simulink model "Motor1conCorrientePrevia"  (R2025b)
settings: Solver=FixedStepDiscrete  StartTime=0.0  StopTime=inf  FixedStep=0.01  RelTol=1e-3  EnableMultiTasking=on
libraries: arduinolib x7, simulink x5, arduinosensorlib x1
settings Model: SimulationMode=external  ExtModeTrigDuration=2  Creator=Vizca  LastModifiedBy=josee
settings SolverCC: AutoInsertRateTranBlk=on
settings OptimizationCC: EnhancedBackFolding=on  PassReuseOutputArgsAs=Individual arguments  ZeroExternalMemoryAtStartup=off  ZeroInternalMemoryAtStartup=off  MaxStackSize=64  OptimizeBlockOrder=speed  DifferentSizesBufferReuse=on  OptimizationCustomize=off  EfficientTunableParamExpr=on
settings DebuggingCC: ParameterTunabilityLossMsg=error
settings HardwareCC: ProdBitPerInt=16.0  ProdBitPerPointer=16.0  ProdBitPerSizeT=16.0  ProdBitPerPtrDiffT=16.0  ProdLargestAtomicFloat=None  ProdWordSize=8.0  ProdHWDeviceType=Atmel->AVR
settings RTWCC: SystemTargetFile=ert.tlc  HardwareBoard=Arduino Uno  TemplateMakefile=ert_default_tmf  Toolchain=Arduino AVR  BuildConfiguration=Faster Runs  Description=Embedded Coder
settings CodeAppCC: ForceParamTrailComments=on  IgnoreCustomStorageClasses=off  OperatorAnnotations=on  SimulinkDataObjDesc=on  SFDataObjDesc=on  InsertBlockDesc=on
settings ERTTargetCC: ExtModeTransport=3.0  ExtModeStaticAlloc=on  ExtModeAutomaticAllocSize=off  ExtModeStaticAllocSize=250.0  ExtModeMexFile=ext_xcp  ExtModeIntrfLevel=Level2 - Open  InlinedParameterPlacement=Hierarchical  SupportContinuousTime=on  SupportVariableSizeSignals=on

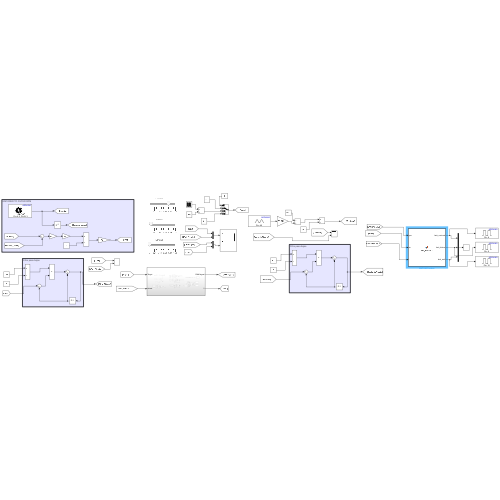
[thumbnail: Simulink's stored preview of the top-level diagram]
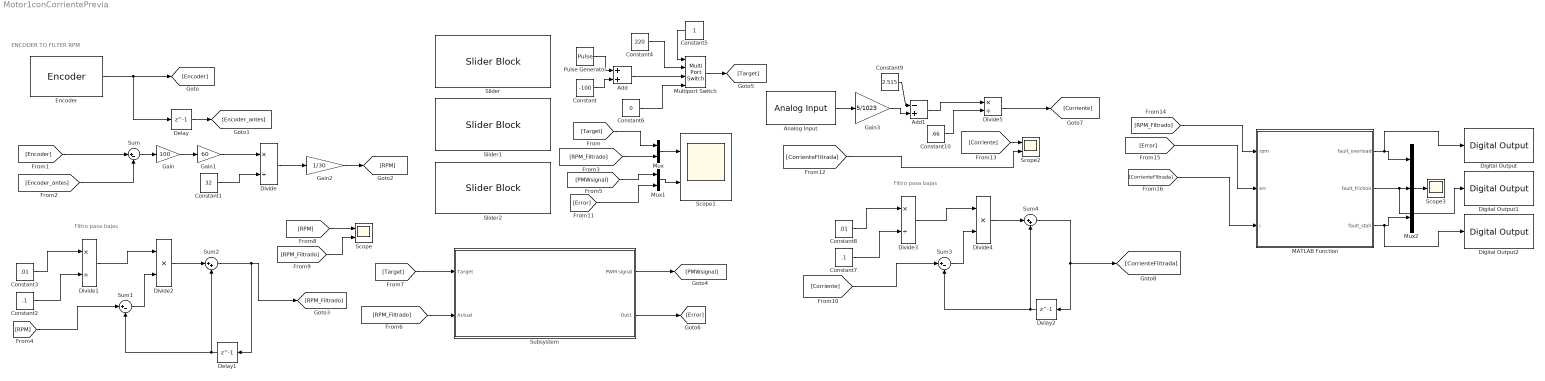
== system Motor1conCorrientePrevia ==
  note: Filtro pasa bajas
  note: ENCODER TO FILTER RPM
  note: Filtro pasa bajas
  Add : Sum
  Add1 : Sum  Inputs=-+
  Analog Input : arduinolib/Analog Input  pinNumber=0  ReadResultsOnly=off  ConversionTriggerSource=Software  ExternalTriggerType=uint32( 0 )  OutputDataType=uint16  EnableConversionCompleteNotify=off  EnableOuputStatus=off  SampleTime=.01  blockPlatform=arduino
  Constant : Constant  Value=-100
  Constant1 : Constant  Value=32
  Constant10 : Constant  Value=.66
  Constant2 : Constant  Value=.1
  Constant3 : Constant  Value=.01
  Constant4 : Constant  Value=220
  Constant5 : Constant
  Constant6 : Constant  Value=0
  Constant7 : Constant  Value=.1
  Constant8 : Constant  Value=.01
  Constant9 : Constant  Value=2.515
  Delay : Delay  DelayLength=1
  Delay1 : Delay  DelayLength=1
  Delay2 : Delay  DelayLength=1
  Digital Output : arduinolib/Digital Output  pinNumber=8  Direction=output  blockPlatform=arduino
  Digital Output1 : arduinolib/Digital Output  pinNumber=9  Direction=output  blockPlatform=arduino
  Digital Output2 : arduinolib/Digital Output  pinNumber=10  Direction=output  blockPlatform=arduino
  Divide{,1,3,5} (4 alike) : Product  Inputs=*/
  Divide2 : Product  Inputs=**
  Divide4 : Product  Inputs=**
  Encoder : arduinosensorlib/Encoder  InputA=2  InputB=3  Mode=No reset  SampleTime=-1
  Gain : Gain  Gain=100
  Gain1 : Gain  Gain=60
  Gain2 : Gain  Gain=1/30
  Gain3 : Gain  Gain=5/1023
  MATLAB Function : MATLAB Function  TreatAsAtomicUnit=on
  Multiport Switch : MultiPortSwitch  SaturateOnIntegerOverflow=off  InputSameDT=off
  Mux : Mux  Inputs=2
  Mux1 : Mux  Inputs=2
  Mux2 : Mux  Inputs=3
  Pulse Generator : DiscretePulseGenerator  PulseType=Time based  Amplitude=200  Period=6  PulseWidth=50
  Scope : Scope  NumInputPorts=2
      settings: ActiveDisplayYMinimum=-33.593749999999993  ActiveDisplayYMaximum=302.34375  DataLoggingVariableName=ScopeData2
  Scope1 : Scope  NumInputPorts=2
      settings: ActiveDisplayYMinimum=-70.450521469116211  ActiveDisplayYMaximum=291.161169052124
  Scope2 : Scope  NumInputPorts=2
      settings: ActiveDisplayYMinimum=-0.066616234284719855  ActiveDisplayYMaximum=0.10203715691215143
  Scope3 : Scope
      settings: ActiveDisplayYMinimum=-0.88521995611242943  ActiveDisplayYMaximum=0.86117560265965387  DataLoggingVariableName=ScopeData3
  Slider : SliderBlock  ScaleMax=1.05
  Slider1 : SliderBlock  ScaleMax=1.05
  Slider2 : SliderBlock  ScaleMax=1.05
  Subsystem : Subsystem
  Sum : Sum  Inputs=|+-
  Sum1 : Sum  Inputs=|+-
  Sum2 : Sum  Inputs=|++
  Sum3 : Sum  Inputs=|+-
  Sum4 : Sum  Inputs=|++
  wires:
  Sum2/1 -> [RPM_Filtrado], Delay1/1
  Constant1/1 -> Divide/2
  Gain/1 -> Gain1/1
  Divide/1 -> Gain2/1
  Encoder/1 -> Delay/1, [Encoder]
  Sum/1 -> Gain/1
  Delay/1 -> [Encoder_antes]
  Gain1/1 -> Divide/1
  [Encoder_antes] -> Sum/2
  [Encoder] -> Sum/1
  Gain2/1 -> [RPM]
  [Target] -> Subsystem/1(Target)
  [RPM_Filtrado] -> Subsystem/2(Actual)
  Subsystem/1(PWM signal) -> [PMWsignal]
  [Target] -> Mux/1
  Mux/1 -> Scope1/1
  [RPM_Filtrado] -> Mux/2
  Sum1/1 -> Divide2/2
  Constant3/1 -> Divide1/1
  Divide2/1 -> Sum2/1
  [RPM] -> Sum1/1
  Delay1/1 -> Sum2/2, Sum1/2
  Constant2/1 -> Divide1/2
  Divide1/1 -> Divide2/1
  Pulse Generator/1 -> Add/1
  Constant/1 -> Add/2
  [RPM] -> Scope/1
  [RPM_Filtrado] -> Scope/2
  [Error] -> Mux1/2
  Mux1/1 -> Scope1/2
  [PMWsignal] -> Mux1/1
  Subsystem/2(Out1) -> [Error]
  Multiport Switch/1 -> [Target]
  Add/1 -> Multiport Switch/3
  Constant4/1 -> Multiport Switch/2
  Constant6/1 -> Multiport Switch/4
  Constant5/1 -> Multiport Switch/1
  Analog Input/1 -> Gain3/1
  Divide3/1 -> Divide4/1
  [Corriente] -> Sum3/1
  Constant8/1 -> Divide3/1
  Delay2/1 -> Sum4/2, Sum3/2
  Sum4/1 -> [CorrienteFlitrada], Delay2/1
  Divide4/1 -> Sum4/1
  Constant7/1 -> Divide3/2
  Sum3/1 -> Divide4/2
  [CorrienteFlitrada] -> Scope2/2
  Gain3/1 -> Add1/2
  Constant9/1 -> Add1/1
  Add1/1 -> Divide5/1
  Constant10/1 -> Divide5/2
  Divide5/1 -> [Corriente]
  [Corriente] -> Scope2/1
  [RPM_Filtrado] -> MATLAB Function/1(rpm)
  [CorrienteFlitrada] -> MATLAB Function/3(i)
  [Error] -> MATLAB Function/2(err)
  MATLAB Function/2(fault_friction) -> Digital Output1/1, Mux2/2
  MATLAB Function/1(fault_overload) -> Digital Output/1, Mux2/1
  MATLAB Function/3(fault_stall) -> Digital Output2/1, Mux2/3
  Mux2/1 -> Scope3/1

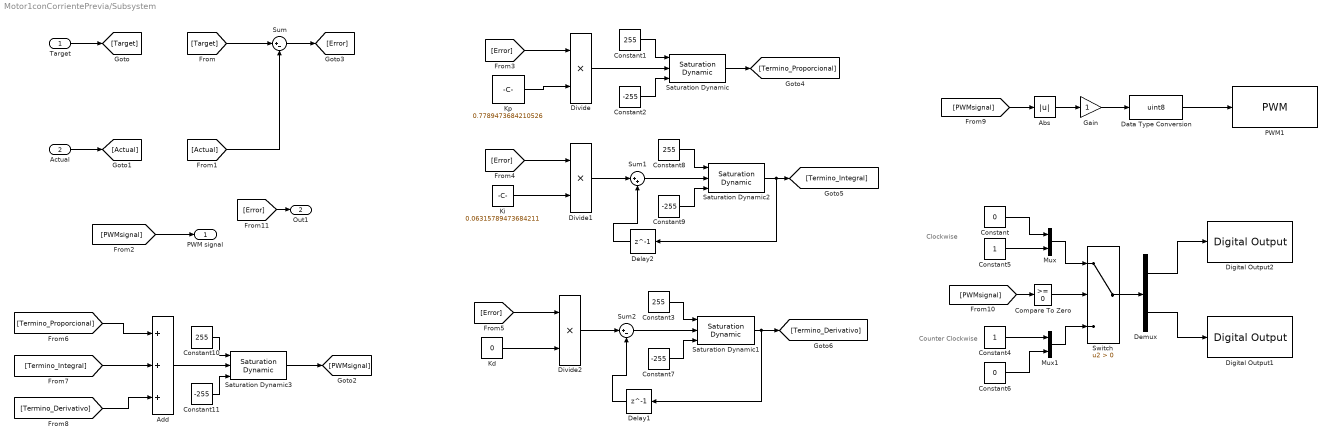
== system Motor1conCorrientePrevia/Subsystem ==
  note: Clockwise
  note: Counter Clockwise
  Target : Inport
  Actual : Inport  Port=2
  Abs : Abs  SaturateOnIntegerOverflow=off
  Add : Sum  Inputs=+++
  Compare To Zero : simulink/Logic and Bit Operations/Compare To Zero  relop=>=  OutDataTypeStr=boolean
  Constant : Constant  Value=0
  Constant{1,3,8,10} (4 alike) : Constant  Value=255
  Constant{2,7,9,11} (4 alike) : Constant  Value=-255
  Constant4 : Constant
  Constant5 : Constant
  Constant6 : Constant  Value=0
  Data Type Conversion : DataTypeConversion  OutMin=0  OutMax=255  OutDataTypeStr=uint8  SaturateOnIntegerOverflow=off  RndMeth=Floor
  Delay1 : Delay  DelayLength=1
  Delay2 : Delay  DelayLength=1
  Demux : Demux  Outputs=2
  Digital Output1 : arduinolib/Digital Output  pinNumber=5  Direction=output  blockPlatform=arduino
  Digital Output2 : arduinolib/Digital Output  pinNumber=4  Direction=output  blockPlatform=arduino
  Divide : Product  Inputs=**
  Divide1 : Product  Inputs=**
  Divide2 : Product  Inputs=**
  Gain : Gain
  Kd : Constant  Value=0
  Ki : Constant  Value=0.06315789473684211
  Kp : Constant  Value=0.7789473684210526
  Mux : Mux  Inputs=2
  Mux1 : Mux  Inputs=2
  PWM1 : arduinolib/PWM  pinNumber=6  frequencyType=Default  desiredFrequency=490.2  achievableFrequency=490.2
  Saturation Dynamic{,1..3} (4 alike) : simulink/Discontinuities/Saturation Dynamic  OutMin=[]  OutMax=[]  OutDataTypeStr=Inherit: Same as second input  OutDataType=fixdt(1, 16)  OutScaling=2^-10  DoSatur=off
  Sum : Sum  Inputs=|+-
  Sum1 : Sum  Inputs=|++
  Sum2 : Sum  Inputs=|+-
  Switch : Switch  Criteria=u2 > Threshold  SaturateOnIntegerOverflow=off  InputSameDT=off
  PWM signal : Outport
  Out1 : Outport  Port=2
  wires:
  Target/1 -> [Target]
  Actual/1 -> [Actual]
  [PWMsignal] -> PWM signal/1
  [Target] -> Sum/1
  [Actual] -> Sum/2
  Sum/1 -> [Error]
  [Error] -> Divide/1
  Kp/1 -> Divide/2
  Divide/1 -> Saturation Dynamic/2
  Ki/1 -> Divide1/2
  [Error] -> Divide1/1
  Divide1/1 -> Sum1/1
  Sum1/1 -> Saturation Dynamic2/2
  Delay1/1 -> Sum2/2
  Divide2/1 -> Sum2/1
  [Error] -> Divide2/1
  Kd/1 -> Divide2/2
  [Termino_Proporcional] -> Add/1
  [Termino_Integral] -> Add/2
  [Termino_Derivativo] -> Add/3
  Add/1 -> Saturation Dynamic3/2
  Data Type Conversion/1 -> PWM1/1
  [PWMsignal] -> Abs/1
  Demux/1 -> Digital Output2/1
  Demux/2 -> Digital Output1/1
  Constant6/1 -> Mux1/2
  Switch/1 -> Demux/1
  Constant/1 -> Mux/1
  Constant5/1 -> Mux/2
  Mux/1 -> Switch/1
  Constant4/1 -> Mux1/1
  Mux1/1 -> Switch/3
  [PWMsignal] -> Compare To Zero/1
  Compare To Zero/1 -> Switch/2
  Saturation Dynamic3/1 -> [PWMsignal]
  Saturation Dynamic/1 -> [Termino_Proporcional]
  Constant1/1 -> Saturation Dynamic/1
  Constant2/1 -> Saturation Dynamic/3
  Constant7/1 -> Saturation Dynamic1/3
  Constant3/1 -> Saturation Dynamic1/1
  Sum2/1 -> Saturation Dynamic1/2
  Saturation Dynamic1/1 -> Delay1/1, [Termino_Derivativo]
  Constant8/1 -> Saturation Dynamic2/1
  Constant9/1 -> Saturation Dynamic2/3
  Saturation Dynamic2/1 -> Delay2/1, [Termino_Integral]
  Delay2/1 -> Sum1/2
  Constant10/1 -> Saturation Dynamic3/1
  Constant11/1 -> Saturation Dynamic3/3
  Abs/1 -> Gain/1
  Gain/1 -> Data Type Conversion/1
  [Error] -> Out1/1

== matlab function Motor1conCorrientePrevia/MATLAB Function ==
  data: rpm input; fault_overload output; err input; i input; fault_friction output; fault_stall output
function [fault_overload, fault_friction, fault_stall] = ...
         fault_detector(rpm, err, i)

% ----- Parámetro del filtro (equivalente a ~100 ms) -----
alpha = 0.95;    
% Mientras más alto = más “parecido a delay de 100 ms”

% ----- Variables persistentes ULTRA pequeñas -----
persistent rpm_d err_d i_d

if isempty(rpm_d)
    rpm_d = rpm;
    err_d = err;
    i_d   = i;
end

% ----- Filtro exponencial (simula retraso sin usar RAM) -----
rpm_d = alpha * rpm_d + (1 - alpha) * rpm;
err_d = alpha * err_d + (1 - alpha) * err;
i_d   = alpha * i_d   + (1 - alpha) * i;

% ----- Márgenes definidos como ±15% respecto al valor filtrado -----
i_max   = i_d   * 1.15;
err_max = err_d * 1.15;
rpm_min = rpm_d * 0.85;

% ----- Inicializar -----
fault_overload = false;
fault_friction = false;
fault_stall    = false;

% ----- Stall -----
if (i > i_max) && (err > err_max) && (rpm < 10)
    fault_stall = true;
end

% ----- Overload -----
if (i > i_max) && (err > err_max) && (rpm < rpm_min)
    fault_overload = true;
end

% ----- Friction -----
if (rpm < rpm_min) && (i > 0.7*i_max) && ~(fault_stall || fault_overload)
    fault_friction = true;
end

end
